simulink model "Realimentacion_VdE"  (Simulink 7.5)
settings: Solver=ode45  StartTime=0.0  StopTime=1  RelTol=1e-3
settings Model: Creator=Nahuek  LastModifiedBy=Nahuek

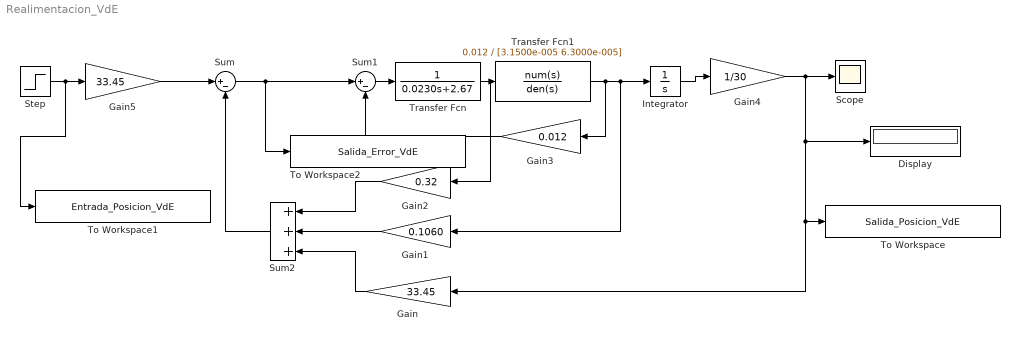
== system Realimentacion_VdE ==
  Display : Display
  Gain : Gain  Gain=33.45  ParameterDataType=fixdt(1, 16)  ParameterScaling=2^0  OutDataType=fixdt(1, 16)  OutScaling=2^0
  Gain1 : Gain  Gain=0.1060  ParameterDataType=fixdt(1, 16)  ParameterScaling=2^0  OutDataType=fixdt(1, 16)  OutScaling=2^0
  Gain2 : Gain  Gain=0.32  ParameterDataType=fixdt(1, 16)  ParameterScaling=2^0  OutDataType=fixdt(1, 16)  OutScaling=2^0
  Gain3 : Gain  Gain=0.012  ParameterDataType=fixdt(1, 16)  ParameterScaling=2^0  OutDataType=fixdt(1, 16)  OutScaling=2^0
  Gain4 : Gain  Gain=1/30  ParameterDataType=fixdt(1, 16)  ParameterScaling=2^0  OutDataType=fixdt(1, 16)  OutScaling=2^0
  Gain5 : Gain  Gain=33.45  ParameterDataType=fixdt(1, 16)  ParameterScaling=2^0  OutDataType=fixdt(1, 16)  OutScaling=2^0
  Integrator : Integrator
  Scope : Scope
      settings: TimeRange=10  YMin=0  YMax=7e+107
  Step : Step  Time=0  SampleTime=0
  Sum : Sum  Inputs=|+-  OutDataType=fixdt(1, 16)  OutScaling=2^0
  Sum1 : Sum  Inputs=|+-  OutDataType=fixdt(1, 16)  OutScaling=2^0
  Sum2 : Sum  Inputs=+++  OutDataType=fixdt(1, 16)  OutScaling=2^0
  To Workspace : ToWorkspace  VariableName=Salida_Posicion_VdE  SampleTime=-1  SaveFormat=Structure With Time
  To Workspace1 : ToWorkspace  VariableName=Entrada_Posicion_VdE  SampleTime=-1  SaveFormat=Structure With Time
  To Workspace2 : ToWorkspace  VariableName=Salida_Error_VdE  SampleTime=-1  SaveFormat=Structure With Time
  Transfer Fcn : TransferFcn  Denominator=[0.0230 2.67]
  Transfer Fcn1 : TransferFcn  Numerator=0.012  Denominator=[3.1500e-005 6.3000e-005]
  wires:
  Transfer Fcn1/1 -> Gain3/1, Integrator/1, Gain1/1
  Transfer Fcn/1 -> Transfer Fcn1/1, Gain2/1
  Gain3/1 -> Sum1/2
  Sum1/1 -> Transfer Fcn/1
  Sum2/1 -> Sum/2
  Gain2/1 -> Sum2/1
  Gain1/1 -> Sum2/2
  Gain/1 -> Sum2/3
  Integrator/1 -> Gain4/1
  Gain4/1 -> Scope/1, Display/1, Gain/1, To Workspace/1
  Gain5/1 -> Sum/1
  Step/1 -> Gain5/1, To Workspace1/1
  Sum/1 -> Sum1/1, To Workspace2/1
